simulink model "PUIO_2"  (R2016b)
settings: Solver=ode45  StartTime=0.0  StopTime=10.0  RelTol=1e-3  EnableMultiTasking=on
values from neighbouring files (symbols this model uses):
  c2 = [0 0 0 1 0 0 0 ... (first row only)    [DPUIO_multipleObservers.m]
  F = A1-K1*C    [DPUIO.m]    (also in DPUIO_LargeGraph.m = A1 - G1*c1; DPUIO_multipleObservers.m = A2 - G1*c2; DPUIOv2.m = A1-G1*c1; DPUIOv3.m = A1 - G1*c1)
  f1Val = 10    [DPUIO_LargeGraph.m]    (also in DPUIO_multipleObservers.m; DPUIOv2.m; DPUIOv3.m; four_cycle.m)
  f2Val = 10    [DPUIO_LargeGraph.m]    (also in DPUIO_multipleObservers.m; DPUIOv2.m; DPUIOv3.m; four_cycle.m)
  f3Val = 10    [DPUIO_LargeGraph.m]    (also in DPUIO_multipleObservers.m; DPUIOv2.m; DPUIOv3.m; four_cycle.m)
  f4Val = 10    [DPUIO_LargeGraph.m]    (also in DPUIO_multipleObservers.m; DPUIOv2.m; DPUIOv3.m; four_cycle.m)
  f5Val = 10    [DPUIO_LargeGraph.m]    (also in DPUIO_multipleObservers.m; DPUIOv2.m; DPUIOv3.m; regularUIOExample.m)
  f6Val = 10    [DPUIO_LargeGraph.m]    (also in DPUIO_multipleObservers.m; DPUIOv2.m; DPUIOv3.m; regularUIOExample.m)
  f7Val = 10    [DPUIO_LargeGraph.m]    (also in DPUIO_multipleObservers.m; DPUIOv2.m; DPUIOv3.m; regularUIOExample.m)
  flt1 = 0    [DPUIO_LargeGraph.m]    (also in DPUIO_multipleObservers.m; DPUIOv2.m; DPUIOv3.m; four_cycle.m)
  flt2 = 0    [DPUIO_LargeGraph.m]    (also in DPUIO_multipleObservers.m; DPUIOv2.m = 1; DPUIOv3.m = 1; four_cycle.m = 1)
  flt3 = 0    [DPUIO_LargeGraph.m]    (also in DPUIO_multipleObservers.m; DPUIOv2.m; DPUIOv3.m; four_cycle.m)
  flt4 = 0    [DPUIO_LargeGraph.m]    (also in DPUIO_multipleObservers.m; DPUIOv2.m; DPUIOv3.m; four_cycle.m)
  flt5 = 1    [DPUIO_LargeGraph.m]    (also in DPUIO_multipleObservers.m; DPUIOv2.m = 0; DPUIOv3.m = 0; regularUIOExample.m = 0)
  flt6 = 0    [DPUIO_LargeGraph.m]    (also in DPUIO_multipleObservers.m; DPUIOv2.m; DPUIOv3.m; regularUIOExample.m)
  flt7 = 0    [DPUIO_LargeGraph.m]    (also in DPUIO_multipleObservers.m; DPUIOv2.m; DPUIOv3.m; regularUIOExample.m)
  G = G1 + A1*N -G1*C*N    [DPUIO.m]    (also in DPUIO_LargeGraph.m = G1 + A1*N - G1*c1*N; DPUIO_multipleObservers.m = G1 + A2*N - G1*c2*N; DPUIOv2.m = G1 + A1*N - G1*c1*N; DPUIOv3.m = G1 + A1*N - G1*c1*N)
  L = Deg-Ag    [DPUIO_LargeGraph.m]    (also in DPUIO_multipleObservers.m; DPUIOv2.m; DPUIOv3.m; four_cycle.m)
  M = eye(size(A))    [DPUIO_LargeGraph.m]    (also in DPUIO_multipleObservers.m; DPUIOv2.m; DPUIOv3.m; four_cycle.m)
  N = E*CEg    [DPUIO.m]    (also in DPUIO_LargeGraph.m; DPUIO_multipleObservers.m; DPUIOv2.m; DPUIOv3.m)
  tf1 = 2    [DPUIO_LargeGraph.m]    (also in DPUIO_multipleObservers.m; DPUIOv2.m; DPUIOv3.m; four_cycle.m)
  tf2 = 2    [DPUIO_LargeGraph.m]    (also in DPUIO_multipleObservers.m; DPUIOv2.m; DPUIOv3.m; four_cycle.m)
  tf3 = 2    [DPUIO_LargeGraph.m]    (also in DPUIO_multipleObservers.m; DPUIOv2.m; DPUIOv3.m; four_cycle.m)
  tf4 = 2    [DPUIO_LargeGraph.m]    (also in DPUIO_multipleObservers.m; DPUIOv2.m; DPUIOv3.m; four_cycle.m)
  tf5 = 2    [DPUIO_LargeGraph.m]    (also in DPUIO_multipleObservers.m; DPUIOv2.m; DPUIOv3.m; regularUIOExample.m)
  tf6 = 5    [DPUIO_LargeGraph.m]    (also in DPUIO_multipleObservers.m; DPUIOv2.m; DPUIOv3.m; regularUIOExample.m)
  tf7 = 7    [DPUIO_LargeGraph.m]    (also in DPUIO_multipleObservers.m; DPUIOv2.m; DPUIOv3.m; regularUIOExample.m)
  x0 = [0 1 1 0 0 0 0]    [DPUIO_multipleObservers.m]    (also in DPUIOv2.m; DPUIOv3.m = [10,1,1,1,1,1,1]; four_cycle.m = [10,1,1,1]; regularUIOExample.m = [0 0 0 0 0 0 0])
settings Model: Creator=sqn4594  LastModifiedBy=samnazari
settings DataIOCC: LimitDataPoints=on  SaveFormat=Array
settings OptimizationCC: LifeSpan=inf
settings DebuggingCC: SolverPrmCheckMsg=warning  FcnCallInpInsideContextMsg=warning  AllowSymbolicDim=off  SFUnexpectedBacktrackingDiag=warning  SFNoUnconditionalDefaultTransitionDiag=warning  SFExecutionAtInitializationDiag=none
settings HardwareCC: ProdBitPerPointer=32  ProdBitPerSizeT=32  ProdBitPerPtrDiffT=32  ProdLargestAtomicFloat=None  ProdIntDivRoundTo=Undefined  ProdEndianess=Unspecified  ProdWordSize=32  ProdHWDeviceType=32-bit Generic
settings ModelReferenceCC: PropagateSignalLabelsOutOfModel=off
settings GRTTargetCC: TargetLangStandard=C89/C90 (ANSI)  GeneratePreprocessorConditionals=Disable all
settings ConfigComp: CovMetricSettings=dw  CovHtmlReporting=on  CovSaveCumulativeToWorkspaceVar=on  CovSaveSingleToWorkspaceVar=on  CovExternalEMLEnable=off

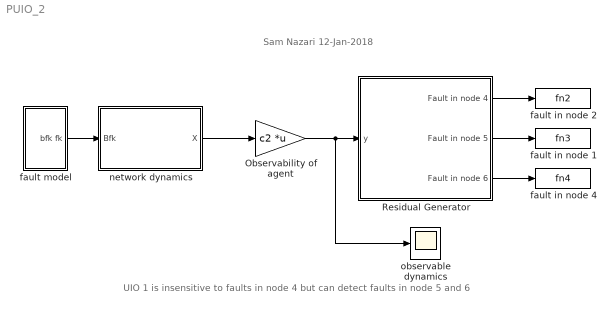
== system PUIO_2 ==
  note: UIO 1 is insensitive to faults in node 4 but can detect faults in node 5 and 6
  note: Sam Nazari
      | 12-Jan-2018
  "Observability of agent " : Gain  Gain=c2  Multiplication=Matrix(K*u)
  Residual Generator : Subsystem
  fault model : Subsystem
  fault in node 1 : ToWorkspace  VariableName=fn3  SaveFormat=Timeseries  SampleTime=-1
  fault in node 2 : ToWorkspace  VariableName=fn2  SaveFormat=Timeseries  SampleTime=-1
  fault in node 4 : ToWorkspace  VariableName=fn4  SaveFormat=Timeseries  SampleTime=-1
  network dynamics : Subsystem
  observable dynamics : Scope
  wires:
  fault model/1(bfk fk) -> network dynamics/1(Bfk)
  network dynamics/1(X) -> "Observability of agent "/1
  "Observability of agent "/1 -> observable dynamics/1, Residual Generator/1(y)
  Residual Generator/1(Fault in node 4) -> fault in node 2/1
  Residual Generator/3(Fault in node 6) -> fault in node 4/1
  Residual Generator/2(Fault in node 5) -> fault in node 1/1

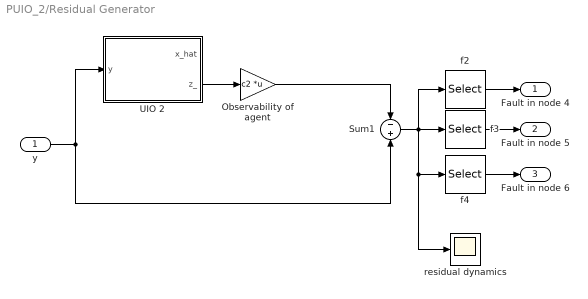
== system PUIO_2/Residual Generator ==
  y : Inport
  "Observability of agent " : Gain  Gain=c2  Multiplication=Matrix(K*u)
  Sum1 : Sum  Inputs=-+
  UIO 2 : Subsystem
  f2 : Selector  InputPortWidth=3  IndexOptions=Index vector (dialog)  Indices=1  OutputSizes=1
  f3 : Selector  InputPortWidth=3  IndexOptions=Index vector (dialog)  Indices=2  OutputSizes=1
  f4 : Selector  InputPortWidth=3  IndexOptions=Index vector (dialog)  Indices=3  OutputSizes=1
  residual dynamics : Scope
  Fault in node 4 : Outport
  Fault in node 5 : Outport  Port=2
  Fault in node 6 : Outport  Port=3
  wires:
  y/1 -> Sum1/2, UIO 2/1(y)
  f2/1 -> Fault in node 4/1
  f4/1 -> Fault in node 6/1
  Sum1/1 -> f2/1, residual dynamics/1, f4/1, f3/1
  f3/1 -> Fault in node 5/1
  UIO 2/2(z_) -> "Observability of agent "/1
  "Observability of agent "/1 -> Sum1/1

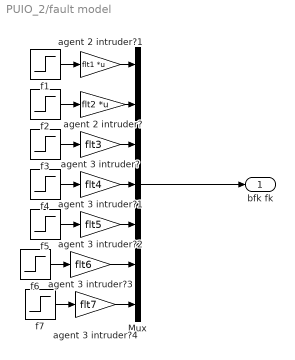
== system PUIO_2/fault model ==
  Mux : Mux  Inputs=7
  agent 2 intruder? : Gain  Gain=flt2  Multiplication=Matrix(K*u)
  agent 2 intruder?1 : Gain  Gain=flt1  Multiplication=Matrix(K*u)
  agent 3 intruder? : Gain  Gain=flt3
  agent 3 intruder?1 : Gain  Gain=flt4
  agent 3 intruder?2 : Gain  Gain=flt5
  agent 3 intruder?3 : Gain  Gain=flt6
  agent 3 intruder?4 : Gain  Gain=flt7
  f1 : Step  After=f1Val  SampleTime=tf1
  f2 : Step  After=f2Val  SampleTime=tf2
  f3 : Step  After=f3Val  SampleTime=tf3
  f4 : Step  After=f4Val  SampleTime=tf4
  f5 : Step  After=f5Val  SampleTime=tf5
  f6 : Step  After=f6Val  SampleTime=tf6
  f7 : Step  After=f7Val  SampleTime=tf7
  bfk fk : Outport
  wires:
  Mux/1 -> bfk fk/1
  f1/1 -> agent 2 intruder?1/1
  f2/1 -> agent 2 intruder?/1
  f3/1 -> agent 3 intruder?/1
  agent 2 intruder?/1 -> Mux/2
  agent 3 intruder?/1 -> Mux/3
  agent 2 intruder?1/1 -> Mux/1
  f4/1 -> agent 3 intruder?1/1
  agent 3 intruder?1/1 -> Mux/4
  agent 3 intruder?2/1 -> Mux/5
  f5/1 -> agent 3 intruder?2/1
  f6/1 -> agent 3 intruder?3/1
  agent 3 intruder?3/1 -> Mux/6
  f7/1 -> agent 3 intruder?4/1
  agent 3 intruder?4/1 -> Mux/7

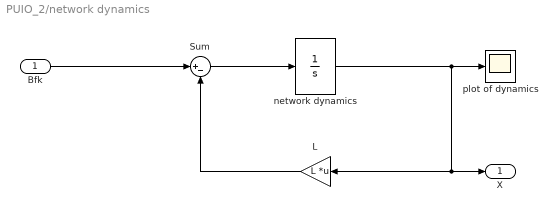
== system PUIO_2/network dynamics ==
  Bfk : Inport
  L : Gain  Gain=L  Multiplication=Matrix(K*u)
  Sum : Sum  Inputs=|+-
  network dynamics : Integrator  InitialCondition=x0
  plot of dynamics : Scope
  X : Outport
  wires:
  Bfk/1 -> Sum/1
  Sum/1 -> network dynamics/1
  network dynamics/1 -> plot of dynamics/1, X/1, L/1
  L/1 -> Sum/2

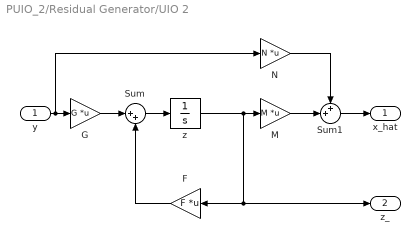
== system PUIO_2/Residual Generator/UIO 2 ==
  y : Inport
  F : Gain  Gain=F  Multiplication=Matrix(K*u)
  G : Gain  Gain=G  Multiplication=Matrix(K*u)
  M : Gain  Gain=M  Multiplication=Matrix(K*u)
  N : Gain  Gain=N  Multiplication=Matrix(K*u)
  Sum : Sum  Inputs=|++
  Sum1 : Sum  Inputs=++|
  z : Integrator
  x_hat : Outport
  z_ : Outport  Port=2
  wires:
  y/1 -> N/1, G/1
  G/1 -> Sum/1
  Sum/1 -> z/1
  F/1 -> Sum/2
  M/1 -> Sum1/2
  N/1 -> Sum1/1
  z/1 -> M/1, z_/1, F/1
  Sum1/1 -> x_hat/1
